simulink model "chargeControlsModel"  (R2023a)
settings: Solver=VariableStepAuto  StartTime=0  StopTime=10000  RelTol=1e-3
model workspace (MAT data in the model file):
  constantCurrent = 1
values from neighbouring files (symbols this model uses):
  c1 = 12    [rcModel.m]
  c2 = 10    [rcModel.m]
  cell = struct    [batteryCell_PANA18650PF.m]
  r0 = 1    [rcModel.m]
  r1 = 10    [rcModel.m]
  r2 = 5    [rcModel.m]
undefined symbols (not defined in the file or in its folder): constantVoltage
libraries: slpidlib x1
settings Model: Creator=deshm  LastModifiedBy=deshm

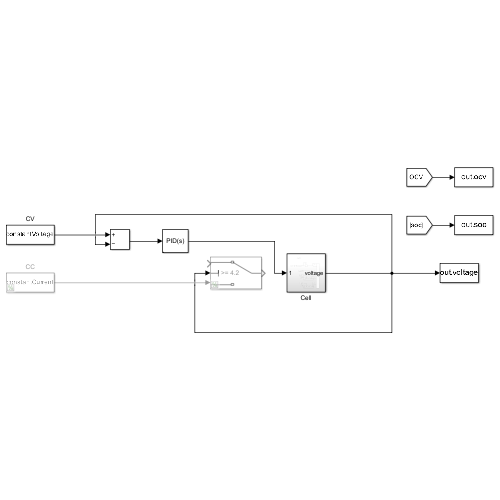
[thumbnail: Simulink's stored preview of the top-level diagram]
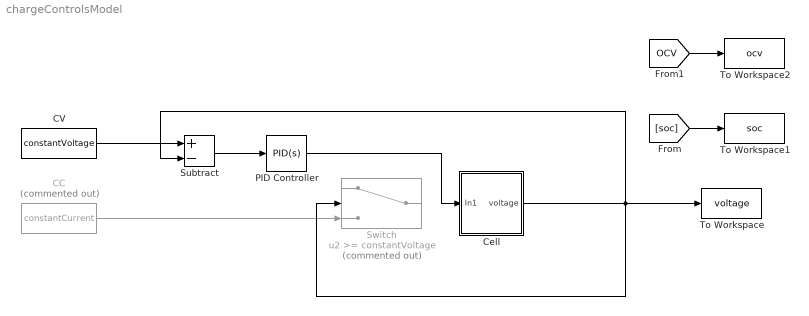
== system chargeControlsModel ==
  CC : Constant  Commented=on  Value=constantCurrent
  CV : Constant  Value=constantVoltage
  Cell : Subsystem
  PID Controller : slpidlib/PID Controller  Controller=PID  Form=Parallel  TimeDomain=Continuous-time  UseExternalTs=off  SampleTime=-1  IntegratorMethod=Forward Euler  FilterMethod=Forward Euler  ControllerParametersSource=internal  P=1  I=1  UseKiTs=off  D=0  N=100  UseFilter=on  TunerSelectOption=Transfer Function Based (PID Tuner App)  InitialConditionSource=internal  InitialConditionForIntegrator=0  InitialConditionForFilter=0  DifferentiatorICPrevScaledInput=0  ExternalReset=none  TrackingMode=off  Kt=1  LimitOutput=off  SatLimitsSource=internal  UpperSaturationLimit=inf  LowerSaturationLimit=-inf  LinearizeAsGain=on  AntiWindupMode=none  Kb=1  LimitIntegrator=off  UpperIntegratorSaturationLimit=inf  LowerIntegratorSaturationLimit=-inf  POutMin=[]  POutMax=[]  IOutMin=[]  IOutMax=[]  DOutMin=[]  DOutMax=[]  NOutMin=[]  NOutMax=[]  SumOutMin=[]  SumOutMax=[]  SaturationOutMin=[]  SaturationOutMax=[]  PParamMin=[]  PParamMax=[]  IParamMin=[]  IParamMax=[]  DParamMin=[]  DParamMax=[]  NParamMin=[]  NParamMax=[]  KbParamMin=[]  KbParamMax=[]  KtParamMin=[]  KtParamMax=[]  KbOutMin=[]  KbOutMax=[]  KtOutMin=[]  KtOutMax=[]  IntegratorOutMin=[]  IntegratorOutMax=[]  FilterOutMin=[]  FilterOutMax=[]  SumI1OutMin=[]  SumI1OutMax=[]  SumI2OutMin=[]  SumI2OutMax=[]  SumI3OutMin=[]  SumI3OutMax=[]  SumI4OutMin=[]  SumI4OutMax=[]  SumDOutMin=[]  SumDOutMax=[]  DifferentiatorOutMin=[]  DifferentiatorOutMax=[]  FilterDiffOutCoefMin=[]  FilterDiffOutCoefMax=[]  ReciprocalOutMin=[]  ReciprocalOutMax=[]  SumDenOutMin=[]  SumDenOutMax=[]  SumNumOutMin=[]  SumNumOutMax=[]  DivideOutMin=[]  DivideOutMax=[]  UdiffTsProdOutMin=[]  UdiffTsProdOutMax=[]  NTsProdOutMin=[]  NTsProdOutMax=[]  UintegralTsProdOutMin=[]  UintegralTsProdOutMax=[]  UngainTsProdOutMin=[]  UngainTsProdOutMax=[]  ClampingZeroOutDataTypeStr=Inherit: Inherit via back propagation  ClampingZeroOutMin=[]  ClampingZeroOutMax=[]  FilterDenConstantOutDataTypeStr=Inherit: Inherit via back propagation  FilterDenConstantOutMin=[]  FilterDenConstantOutMax=[]  PCopyOutDataTypeStr=Inherit: Inherit via back propagation  PCopyOutMin=[]  PCopyOutMax=[]  NCopyOutDataTypeStr=Inherit: Inherit via back propagation  NCopyOutMin=[]  NCopyOutMax=[]  IntegratorContinuousStateAttributes=''  IntegratorStateMustResolveToSignalObject=off  IntegratorRTWStateStorageClass=Auto  FilterContinuousStateAttributes=''  FilterStateMustResolveToSignalObject=off  FilterRTWStateStorageClass=Auto  ParallelPVariant=InternalParameters  IdealPVariant=Disabled  IVariant=InternalParameters  DVariant=InternalParameters  IntegratorVariant=Continuous  SatVariant=Disabled  AWVariant=Passthrough  PCopyVariant=Disabled  TRVariant=Disabled  FdbkBlocksVariant=Forward  IdealPFdbkVariant=Disabled  SatFdbkVariant=Disabled  DerivativeFilterVariant=ContFilter  NVariant=InternalParameters  NCopyVariant=Disabled  FilterICVariant=InternalICsFilter  IntegratorICVariant=InternalICs  ExternalResetVariant=Disabled  TRSumVariant=Passthrough  SumFdbkVariant=Disabled  SumVariant=Sum_PID  TsampFilterVariant=InternalTs  TsampNgainVariant=Passthrough  TsampIntegralVariant=Disabled_SignalSpec  ExternalSaturationOutDataTypeStr=Inherit: Same as second input
  Subtract : Sum  Inputs=+-
  Switch : Switch  Commented=on  Threshold=constantVoltage  SaturateOnIntegerOverflow=off  InputSameDT=off
  To Workspace : ToWorkspace  VariableName=voltage  SaveFormat=Timeseries  SampleTime=-1
  To Workspace1 : ToWorkspace  VariableName=soc  SaveFormat=Timeseries  SampleTime=-1
  To Workspace2 : ToWorkspace  VariableName=ocv  SaveFormat=Timeseries  SampleTime=-1
  wires:
  CC/1 -> Switch/3
  CV/1 -> Subtract/1
  Cell/1(voltage) -> To Workspace/1, Subtract/2, Switch/2
  Subtract/1 -> PID Controller/1
  [soc] -> To Workspace1/1
  [OCV] -> To Workspace2/1
  PID Controller/1 -> Cell/1(In1)

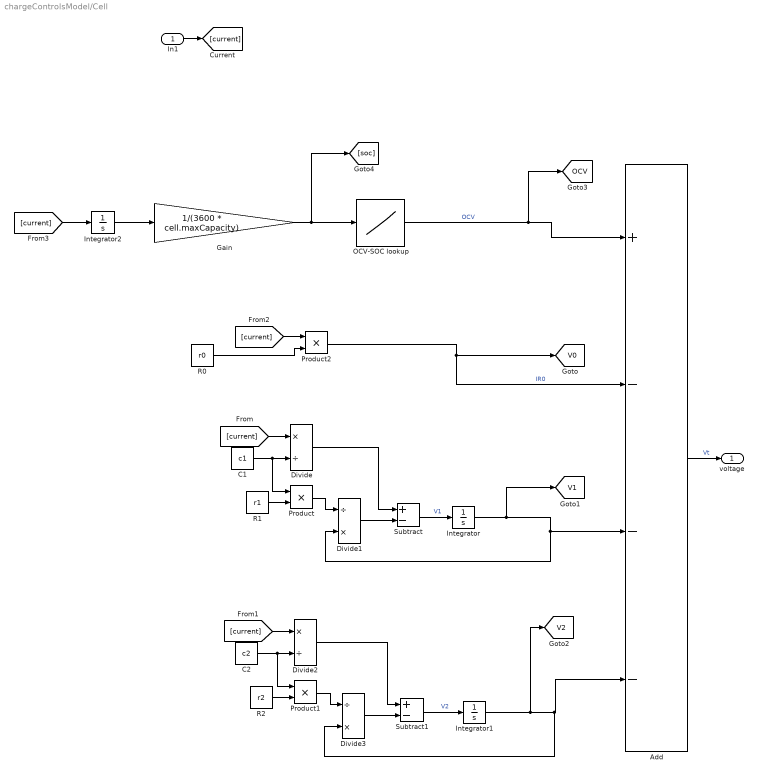
== system chargeControlsModel/Cell ==
  In1 : Inport
  Add : Sum  Inputs=+---
  C1 : Constant  Value=c1
  C2 : Constant  Value=c2
  Divide : Product  Inputs=*/
  Divide1 : Product  Inputs=/*
  Divide2 : Product  Inputs=*/
  Divide3 : Product  Inputs=/*
  Gain : Gain  Gain=1/(3600 * cell.maxCapacity)
  Integrator : Integrator
  Integrator1 : Integrator
  Integrator2 : Integrator
  OCV-SOC lookup : Lookup_n-D  NumberOfTableDimensions=1  BreakpointsForDimension1=cell.soc  Table=cell.ocv.charge  InternalRulePriority=Speed  RndMeth=Simplest
  Product : Product
  Product1 : Product
  Product2 : Product
  R0 : Constant  Value=r0
  R1 : Constant  Value=r1
  R2 : Constant  Value=r2
  Subtract : Sum  Inputs=+-
  Subtract1 : Sum  Inputs=+-
  voltage : Outport
  tag scope: OCV=global, V0=global, V1=global, V2=global
  wires:
  Integrator/1 -> [V1], Divide1/2, Add/3
  OCV-SOC lookup/1 -> [OCV], Add/1  "OCV"
  [current] -> Divide/1
  C2/1 -> Divide2/2, Product1/1
  Divide3/1 -> Subtract1/2
  Subtract1/1 -> Integrator1/1  "V2"
  [current] -> Integrator2/1
  Divide/1 -> Subtract/1
  C1/1 -> Divide/2, Product/1
  R0/1 -> Product2/2
  Divide2/1 -> Subtract1/1
  Subtract/1 -> Integrator/1  "V1"
  R1/1 -> Product/2
  Integrator1/1 -> [V2], Divide3/2, Add/4
  Product1/1 -> Divide3/1
  [current] -> Product2/1
  Gain/1 -> [soc], OCV-SOC lookup/1
  Add/1 -> voltage/1  "Vt"
  Product2/1 -> Add/2, [V0]  "IR0"
  Integrator2/1 -> Gain/1
  In1/1 -> [current]
  [current] -> Divide2/1
  R2/1 -> Product1/2
  Product/1 -> Divide1/1
  Divide1/1 -> Subtract/2
